simulink library "TMCA_lib"  (Simulink 7.5)
settings: Solver=ode45  StartTime=0.0  StopTime=10.0  RelTol=1e-3
values from neighbouring files (symbols this model uses):
  pTMCA_A_BatCurrHi_C = Simulink.Parameter    [TMCA_par.m]
  pTMCA_A_BatCurrLo_C = Simulink.Parameter    [TMCA_par.m]
  pTMCA_bool_ACPtcConfig_C = Simulink.Parameter    [TMCA_par.m]
  pTMCA_bool_BatCoolACReqCtrl_C = Simulink.Parameter    [TMCA_par.m]
  pTMCA_bool_BatCoolACReqEnbl_C = Simulink.Parameter    [TMCA_par.m]
  pTMCA_bool_BatCoolEnbl_C = Simulink.Parameter    [TMCA_par.m]
  pTMCA_bool_BatHeatEnbl_C = Simulink.Parameter    [TMCA_par.m]
  pTMCA_bool_ChrgrValveCtrl_C = Simulink.Parameter    [TMCA_par.m]
  pTMCA_bool_ChrgrValveEnbl_C = Simulink.Parameter    [TMCA_par.m]
  pTMCA_bool_FanCtrlEnbl = Simulink.Parameter    [TMCA_par.m]
  pTMCA_bool_FanCtrlSwitch = Simulink.Parameter    [TMCA_par.m]
  pTMCA_bool_Mot1PmpEnbl_C = Simulink.Parameter    [TMCA_par.m]
  pTMCA_bool_Mot2PmpEnbl_C = Simulink.Parameter    [TMCA_par.m]
  pTMCA_bool_MotValveCtrl_C = Simulink.Parameter    [TMCA_par.m]
  pTMCA_bool_MotValveEnbl_C = Simulink.Parameter    [TMCA_par.m]
  pTMCA_bool_TMCoolEnbl_C = Simulink.Parameter    [TMCA_par.m]
  pTMCA_bool_WtrPmpCoolEnbl_C = Simulink.Parameter    [TMCA_par.m]
  pTMCA_bool_WtrPmpHeatEnbl_C = Simulink.Parameter    [TMCA_par.m]
  pTMCA_cnt_ACHeatTime_CUR = Simulink.Parameter    [TMCA_par.m]
  pTMCA_cnt_DCTempTime_CUR = Simulink.Parameter    [TMCA_par.m]
  pTMCA_cnt_TimeDwnLim_C = Simulink.Parameter    [TMCA_par.m]
  pTMCA_cnt_TimeUpLim_C = Simulink.Parameter    [TMCA_par.m]
  pTMCA_degC_AmbHiTempDisply_C = Simulink.Parameter    [TMCA_par.m]
  pTMCA_degC_BatCoolAmbHiTemp_C = Simulink.Parameter    [TMCA_par.m]
  pTMCA_degC_BatCoolAmbLoTemp_C = Simulink.Parameter    [TMCA_par.m]
  pTMCA_degC_BatCoolHiTemp_C = Simulink.Parameter    [TMCA_par.m]
  pTMCA_degC_BatCoolLoTemp_C = Simulink.Parameter    [TMCA_par.m]
  pTMCA_degC_BatHiTempDisply_C = Simulink.Parameter    [TMCA_par.m]
  pTMCA_degC_BatMaxT_CUR = Simulink.Parameter    [TMCA_par.m]
  pTMCA_degC_BatMaxTHiThd_C = Simulink.Parameter    [TMCA_par.m]
  pTMCA_degC_BatMaxTLoThd_C = Simulink.Parameter    [TMCA_par.m]
  pTMCA_degC_ChrgrHiTThd_C = Simulink.Parameter    [TMCA_par.m]
  pTMCA_degC_ChrgrLoTThd_C = Simulink.Parameter    [TMCA_par.m]
  pTMCA_degC_ChrgrTThd_CUR = Simulink.Parameter    [TMCA_par.m]
  pTMCA_degC_DcDcHiTThd_C = Simulink.Parameter    [TMCA_par.m]
  pTMCA_degC_DcDcLoTThd_C = Simulink.Parameter    [TMCA_par.m]
  pTMCA_degC_DcDcTThd_CUR = Simulink.Parameter    [TMCA_par.m]
  pTMCA_degC_MotWtrHiTThd_C = Simulink.Parameter    [TMCA_par.m]
  pTMCA_degC_MotWtrLoTThd_C = Simulink.Parameter    [TMCA_par.m]
  pTMCA_degC_MotWtrMaxTThd_C = Simulink.Parameter    [TMCA_par.m]
  pTMCA_degC_MotWtrMinTThd_C = Simulink.Parameter    [TMCA_par.m]
  pTMCA_pct_ACHeatPTCPWM_CUR = Simulink.Parameter    [TMCA_par.m]
  pTMCA_pct_BatWtrPmpPWM_CUR = Simulink.Parameter    [TMCA_par.m]
  pTMCA_pct_ChrgrWtrPmpPWM_CUR = Simulink.Parameter    [TMCA_par.m]
  pTMCA_pct_DcDcWtrPmpPWM_CUR = Simulink.Parameter    [TMCA_par.m]
  pTMCA_pct_DCHeatPTCPWM_CUR = Simulink.Parameter    [TMCA_par.m]
  pTMCA_pct_HeatPTCCtrl_C = Simulink.Parameter    [TMCA_par.m]
  pTMCA_pct_HeatPTCEnbl_C = Simulink.Parameter    [TMCA_par.m]
  pTMCA_pct_HeatrOffVal_C = Simulink.Parameter    [TMCA_par.m]
  pTMCA_pct_Mot1PmpPWMCtrl_C = Simulink.Parameter    [TMCA_par.m]
  pTMCA_pct_Mot2PmpPWMCtrl_C = Simulink.Parameter    [TMCA_par.m]
  pTMCA_pct_MotWtrPmpMaxSpd_C = Simulink.Parameter    [TMCA_par.m]
  pTMCA_pct_MotWtrPmpMinSpd_C = Simulink.Parameter    [TMCA_par.m]
  pTMCA_pct_MotWtrPmpNormSpd_C = Simulink.Parameter    [TMCA_par.m]
  pTMCA_pct_MotWtrPmpZeroSpd_C = Simulink.Parameter    [TMCA_par.m]
  pTMCA_pct_WtrPmpCoolCtrl_C = Simulink.Parameter    [TMCA_par.m]
  pTMCA_pct_WtrPmpHeatCtrl_C = Simulink.Parameter    [TMCA_par.m]
  pTMCA_s_ACDisChrgTimout_C = Simulink.Parameter    [TMCA_par.m]
  pTMCA_s_TFilSampleTi_C = Simulink.Parameter    [TMCA_par.m]
  pTMCA_st_AirCdnOn_C = Simulink.Parameter    [TMCA_par.m]
undefined symbols (not defined in the file or in its folder): AirCdnFanReqTyp, ChrgActStsTyp, MCUCoolReqTyp, p_bool_False_M, p_bool_True_M, PUDCoorrStsTyp
libraries: BaseOperationLib_Browser x197, PES_CZ_FAW x3, simulink x1
(part 2 of 2)

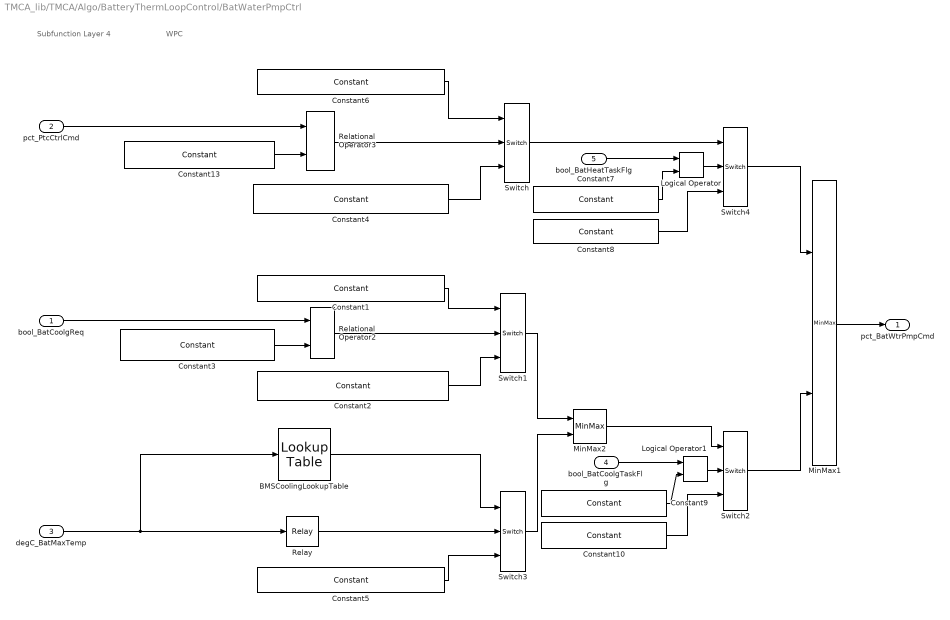
== system TMCA_lib/TMCA/Algo/BatteryThermLoopControl/BatWaterPmpCtrl ==
  note: WPC
  note: Subfunction Layer 4
  bool_BatCoolgReq : Inport  OutDataType=fixdt(1, 16)  OutScaling=2^0
  pct_PtcCtrlCmd : Inport  Port=2  OutDataType=fixdt(1, 16)  OutScaling=2^0
  degC_BatMaxTemp : Inport  Port=3  OutDataType=fixdt(1, 16)  OutScaling=2^0
  bool_BatCoolgTaskFlg : Inport  Port=4  OutDataType=fixdt(1, 16)  OutScaling=2^0
  bool_BatHeatTaskFlg : Inport  Port=5  OutDataType=fixdt(1, 16)  OutScaling=2^0
  BMSCoolingLookupTable : BaseOperationLib_Browser/Lookup Tables Changed/Lookup Table  InputValues=pTMCA_degC_BatMaxT_CUR  Table=pTMCA_pct_BatWtrPmpPWM_CUR  LookUpMeth=Interpolation-Use End Values  OutMin=[]  OutMax=[]  OutDataType=fixdt(1, 16)  OutScaling=2^0  OutDataTypeStr=Inherit: Inherit via back propagation  SaturateOnIntegerOverflow=on
      settings: AttributesFormatString=X:%<InputValues>\nTAB:%<Table>
  Constant1 : BaseOperationLib_Browser/Sources&Sinks/Constant  Value=pTMCA_pct_MotWtrPmpZeroSpd_C  OutMin=[]  OutMax=[]  OutDataType=fixdt(1, 16)  ConRadixGroup=Use specified scaling  OutScaling=2^0  OutDataTypeStr=Inherit: Inherit from 'Constant value'
  Constant10 : BaseOperationLib_Browser/Sources&Sinks/Constant  Value=pTMCA_pct_WtrPmpCoolCtrl_C  OutMin=[]  OutMax=[]  OutDataType=fixdt(1, 16)  ConRadixGroup=Use specified scaling  OutScaling=2^0  OutDataTypeStr=Inherit: Inherit from 'Constant value'
  Constant13 : BaseOperationLib_Browser/Sources&Sinks/Constant  Value=pTMCA_pct_HeatrOffVal_C  OutMin=[]  OutMax=[]  OutDataType=fixdt(1, 16)  ConRadixGroup=Use specified scaling  OutScaling=2^0  OutDataTypeStr=Inherit: Inherit from 'Constant value'
  Constant2 : BaseOperationLib_Browser/Sources&Sinks/Constant  Value=pTMCA_pct_MotWtrPmpMaxSpd_C  OutMin=[]  OutMax=[]  OutDataType=Enum: EgyCoorrStsTyp  ConRadixGroup=Best Precision: Vector-wise  OutScaling=[]  OutDataTypeStr=Inherit: Inherit from 'Constant value'
  Constant3 : BaseOperationLib_Browser/Sources&Sinks/Constant  Value=p_bool_False_M  OutMin=[]  OutMax=[]  OutDataType=fixdt(1, 16)  ConRadixGroup=Use specified scaling  OutScaling=2^0  OutDataTypeStr=Inherit: Inherit from 'Constant value'
  Constant4 : BaseOperationLib_Browser/Sources&Sinks/Constant  Value=pTMCA_pct_MotWtrPmpMaxSpd_C  OutMin=[]  OutMax=[]  OutDataType=Enum: EgyCoorrStsTyp  ConRadixGroup=Best Precision: Vector-wise  OutScaling=[]  OutDataTypeStr=Inherit: Inherit from 'Constant value'
  Constant5 : BaseOperationLib_Browser/Sources&Sinks/Constant  Value=pTMCA_pct_MotWtrPmpZeroSpd_C  OutMin=[]  OutMax=[]  OutDataType=fixdt(1, 16)  ConRadixGroup=Use specified scaling  OutScaling=2^0  OutDataTypeStr=Inherit: Inherit from 'Constant value'
  Constant6 : BaseOperationLib_Browser/Sources&Sinks/Constant  Value=pTMCA_pct_MotWtrPmpZeroSpd_C  OutMin=[]  OutMax=[]  OutDataType=fixdt(1, 16)  ConRadixGroup=Use specified scaling  OutScaling=2^0  OutDataTypeStr=Inherit: Inherit from 'Constant value'
  Constant7 : BaseOperationLib_Browser/Sources&Sinks/Constant  Value=pTMCA_bool_WtrPmpHeatEnbl_C  OutMin=[]  OutMax=[]  OutDataType=fixdt(1, 16)  ConRadixGroup=Use specified scaling  OutScaling=2^0  OutDataTypeStr=Inherit: Inherit from 'Constant value'
  Constant8 : BaseOperationLib_Browser/Sources&Sinks/Constant  Value=pTMCA_pct_WtrPmpHeatCtrl_C  OutMin=[]  OutMax=[]  OutDataType=fixdt(1, 16)  ConRadixGroup=Use specified scaling  OutScaling=2^0  OutDataTypeStr=Inherit: Inherit from 'Constant value'
  Constant9 : BaseOperationLib_Browser/Sources&Sinks/Constant  Value=pTMCA_bool_WtrPmpCoolEnbl_C  OutMin=[]  OutMax=[]  OutDataType=fixdt(1, 16)  ConRadixGroup=Use specified scaling  OutScaling=2^0  OutDataTypeStr=Inherit: Inherit from 'Constant value'
  Logical Operator : BaseOperationLib_Browser/Logic Operations Changed/Logical Operator  Operator=AND  Inputs=2  AllPortsSameDT=on  OutDataTypeMode=Specify via dialog  LogicDataType=PDT_Bool  OutDataTypeStr=PDT_Bool
  Logical Operator1 : BaseOperationLib_Browser/Logic Operations Changed/Logical Operator  Operator=AND  Inputs=2  AllPortsSameDT=on  OutDataTypeMode=Specify via dialog  LogicDataType=PDT_Bool  OutDataTypeStr=PDT_Bool
  MinMax1 : BaseOperationLib_Browser/Math Operations Changed/MinMax  Function=max  Inputs=2  InputSameDT=on  OutMin=[]  OutMax=[]  OutDataType=fixdt(1, 16)  OutScaling=2^0  SaturateOnIntegerOverflow=on
  MinMax2 : BaseOperationLib_Browser/Math Operations Changed/MinMax  Function=max  Inputs=2  InputSameDT=on  OutMin=[]  OutMax=[]  OutDataType=fixdt(1, 16)  OutScaling=2^0  SaturateOnIntegerOverflow=on
  Relational Operator2 : BaseOperationLib_Browser/Logic Operations Changed/Relational Operator  Operator===  InputSameDT=on  LogicOutDataTypeMode=Specify via dialog  LogicDataType=PDT_Bool  OutDataTypeStr=PDT_Bool
  Relational Operator3 : BaseOperationLib_Browser/Logic Operations Changed/Relational Operator  Operator===  InputSameDT=on  LogicOutDataTypeMode=Specify via dialog  LogicDataType=PDT_Bool  OutDataTypeStr=PDT_Bool
  Relay : BaseOperationLib_Browser/Discontinuities Changed/Relay  OnSwitchValue=pTMCA_degC_BatMaxTHiThd_C  OffSwitchValue=pTMCA_degC_BatMaxTLoThd_C  OnOutputValue=p_bool_True_M  OffOutputValue=p_bool_False_M  OutMin=[]  OutMax=[]  OutDataType=fixdt(1, 16)  ConRadixGroup=Use specified scaling  OutScaling=2^0  OutDataTypeStr=Inherit: Inherit via back propagation
      settings: AttributesFormatString=%<OnSwitchValue> OnOut %<OnOutputValue>\n%<OffSwitchValue> OffOut %<OffOutputValue>
  Switch{,1..4} (5 alike) : BaseOperationLib_Browser/Signal Routing Changed/Switch  Criteria=u2 ~= 0  Threshold=1  InputSameDT=on  OutMin=[]  OutMax=[]  OutDataType=fixdt(1,16,0)  OutScaling=[]  SaturateOnIntegerOverflow=on
  pct_BatWtrPmpCmd : Outport  OutDataType=fixdt(1, 16)  OutScaling=2^0
  wires:
  Constant2/1 -> Switch1/3
  Constant1/1 -> Switch1/1
  Relational Operator2/1 -> Switch1/2
  bool_BatCoolgReq/1 -> Relational Operator2/1
  Constant3/1 -> Relational Operator2/2
  Constant6/1 -> Switch/1
  Constant4/1 -> Switch/3
  Relational Operator3/1 -> Switch/2
  Constant13/1 -> Relational Operator3/2
  pct_PtcCtrlCmd/1 -> Relational Operator3/1
  Switch/1 -> Switch4/1
  Relay/1 -> Switch3/2
  degC_BatMaxTemp/1 -> Relay/1, BMSCoolingLookupTable/1
  BMSCoolingLookupTable/1 -> Switch3/1
  Constant5/1 -> Switch3/3
  Switch1/1 -> MinMax2/1
  Switch3/1 -> MinMax2/2
  MinMax2/1 -> Switch2/1
  Switch4/1 -> MinMax1/1
  Switch2/1 -> MinMax1/2
  MinMax1/1 -> pct_BatWtrPmpCmd/1
  Logical Operator/1 -> Switch4/2
  bool_BatHeatTaskFlg/1 -> Logical Operator/1
  Logical Operator1/1 -> Switch2/2
  bool_BatCoolgTaskFlg/1 -> Logical Operator1/1
  Constant7/1 -> Logical Operator/2
  Constant8/1 -> Switch4/3
  Constant9/1 -> Logical Operator1/2
  Constant10/1 -> Switch2/3

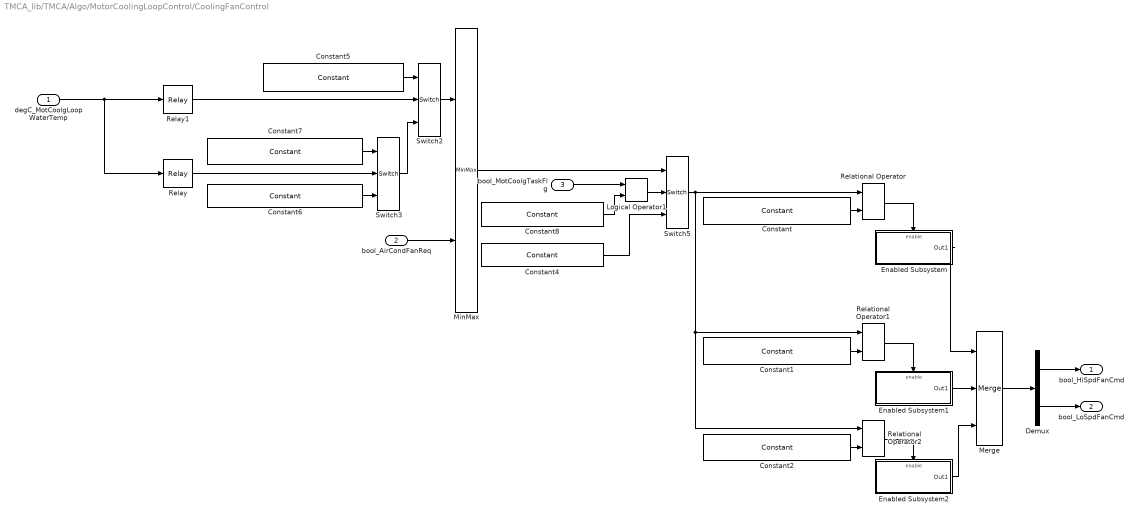
== system TMCA_lib/TMCA/Algo/MotorCoolingLoopControl/CoolingFanControl ==
  degC_MotCoolgLoopWaterTemp : Inport  OutDataType=fixdt(1, 16)  OutScaling=2^0
  bool_AirCondFanReq : Inport  Port=2  OutDataType=fixdt(1, 16)  OutScaling=2^0
  bool_MotCoolgTaskFlg : Inport  Port=3  OutDataType=fixdt(1, 16)  OutScaling=2^0
  Constant : BaseOperationLib_Browser/Sources&Sinks/Constant  Value=uint8(AirCdnFanReqTyp.ACF_HI_SPD)  OutMin=[]  OutMax=[]  OutDataType=fixdt(1, 16)  ConRadixGroup=Use specified scaling  OutScaling=2^0  OutDataTypeStr=Inherit: Inherit from 'Constant value'
  Constant1 : BaseOperationLib_Browser/Sources&Sinks/Constant  Value=uint8(AirCdnFanReqTyp.ACF_LO_SPD)  OutMin=[]  OutMax=[]  OutDataType=fixdt(1, 16)  ConRadixGroup=Use specified scaling  OutScaling=2^0  OutDataTypeStr=Inherit: Inherit from 'Constant value'
  Constant2 : BaseOperationLib_Browser/Sources&Sinks/Constant  Value=uint8(AirCdnFanReqTyp.ACF_OFF)  OutMin=[]  OutMax=[]  OutDataType=fixdt(1, 16)  ConRadixGroup=Use specified scaling  OutScaling=2^0  OutDataTypeStr=Inherit: Inherit from 'Constant value'
  Constant4 : BaseOperationLib_Browser/Sources&Sinks/Constant  Value=pTMCA_bool_FanCtrlSwitch  OutMin=[]  OutMax=[]  OutDataType=fixdt(1, 16)  ConRadixGroup=Use specified scaling  OutScaling=2^0  OutDataTypeStr=Inherit: Inherit from 'Constant value'
  Constant5 : BaseOperationLib_Browser/Sources&Sinks/Constant  Value=uint8(AirCdnFanReqTyp.ACF_HI_SPD)  OutMin=[]  OutMax=[]  OutDataType=fixdt(1, 16)  ConRadixGroup=Use specified scaling  OutScaling=2^0  OutDataTypeStr=Inherit: Inherit from 'Constant value'
  Constant6 : BaseOperationLib_Browser/Sources&Sinks/Constant  Value=uint8(AirCdnFanReqTyp.ACF_OFF)  OutMin=[]  OutMax=[]  OutDataType=fixdt(1, 16)  ConRadixGroup=Use specified scaling  OutScaling=2^0  OutDataTypeStr=Inherit: Inherit from 'Constant value'
  Constant7 : BaseOperationLib_Browser/Sources&Sinks/Constant  Value=uint8(AirCdnFanReqTyp.ACF_LO_SPD)  OutMin=[]  OutMax=[]  OutDataType=fixdt(1, 16)  ConRadixGroup=Use specified scaling  OutScaling=2^0  OutDataTypeStr=Inherit: Inherit from 'Constant value'
  Constant8 : BaseOperationLib_Browser/Sources&Sinks/Constant  Value=pTMCA_bool_FanCtrlEnbl  OutMin=[]  OutMax=[]  OutDataType=fixdt(1, 16)  ConRadixGroup=Use specified scaling  OutScaling=2^0  OutDataTypeStr=Inherit: Inherit from 'Constant value'
  Demux : Demux  Outputs=2
  Enabled Subsystem : Subsystem  TreatAsAtomicUnit=on
  Enabled Subsystem1 : Subsystem  TreatAsAtomicUnit=on
  Enabled Subsystem2 : Subsystem  TreatAsAtomicUnit=on
  Logical Operator1 : BaseOperationLib_Browser/Logic Operations Changed/Logical Operator  Operator=AND  Inputs=2  AllPortsSameDT=on  OutDataTypeMode=Specify via dialog  LogicDataType=PDT_Bool  OutDataTypeStr=PDT_Bool
  Merge : Merge  Inputs=3
  MinMax : BaseOperationLib_Browser/Math Operations Changed/MinMax  Function=max  Inputs=2  InputSameDT=on  OutMin=[]  OutMax=[]  OutDataTypeMode=uint8  OutDataType=fixdt(1, 16)  OutScaling=2^0  OutDataTypeStr=uint8  SaturateOnIntegerOverflow=on
  Relational Operator : BaseOperationLib_Browser/Logic Operations Changed/Relational Operator  Operator===  InputSameDT=on  LogicOutDataTypeMode=Specify via dialog  LogicDataType=PDT_Bool  OutDataTypeStr=PDT_Bool
  Relational Operator1 : BaseOperationLib_Browser/Logic Operations Changed/Relational Operator  Operator===  InputSameDT=on  LogicOutDataTypeMode=Specify via dialog  LogicDataType=PDT_Bool  OutDataTypeStr=PDT_Bool
  Relational Operator2 : BaseOperationLib_Browser/Logic Operations Changed/Relational Operator  Operator===  InputSameDT=on  LogicOutDataTypeMode=Specify via dialog  LogicDataType=PDT_Bool  OutDataTypeStr=PDT_Bool
  Relay : BaseOperationLib_Browser/Discontinuities Changed/Relay  OnSwitchValue=pTMCA_degC_MotWtrHiTThd_C  OffSwitchValue=pTMCA_degC_MotWtrLoTThd_C  OnOutputValue=p_bool_True_M  OffOutputValue=p_bool_False_M  OutMin=[]  OutMax=[]  OutDataType=fixdt(1, 16)  ConRadixGroup=Use specified scaling  OutScaling=2^0  OutDataTypeStr=Inherit: Inherit via back propagation
      settings: AttributesFormatString=%<OnSwitchValue> OnOut %<OnOutputValue>\n%<OffSwitchValue> OffOut %<OffOutputValue>
  Relay1 : BaseOperationLib_Browser/Discontinuities Changed/Relay  OnSwitchValue=pTMCA_degC_MotWtrMaxTThd_C  OffSwitchValue=pTMCA_degC_MotWtrMinTThd_C  OnOutputValue=p_bool_True_M  OffOutputValue=p_bool_False_M  OutMin=[]  OutMax=[]  OutDataType=fixdt(1, 16)  ConRadixGroup=Use specified scaling  OutScaling=2^0  OutDataTypeStr=Inherit: Inherit via back propagation
      settings: AttributesFormatString=%<OnSwitchValue> OnOut %<OnOutputValue>\n%<OffSwitchValue> OffOut %<OffOutputValue>
  Switch2 : BaseOperationLib_Browser/Signal Routing Changed/Switch  Criteria=u2 ~= 0  Threshold=1  InputSameDT=on  OutMin=[]  OutMax=[]  OutDataType=fixdt(1,16,0)  OutScaling=[]  SaturateOnIntegerOverflow=on
  Switch3 : BaseOperationLib_Browser/Signal Routing Changed/Switch  Criteria=u2 ~= 0  Threshold=1  InputSameDT=on  OutMin=[]  OutMax=[]  OutDataType=fixdt(1,16,0)  OutScaling=[]  SaturateOnIntegerOverflow=on
  Switch5 : BaseOperationLib_Browser/Signal Routing Changed/Switch  Criteria=u2 ~= 0  Threshold=1  InputSameDT=on  OutMin=[]  OutMax=[]  OutDataType=fixdt(1,16,0)  OutScaling=[]  SaturateOnIntegerOverflow=on
  bool_HiSpdFanCmd : Outport  OutDataType=fixdt(1, 16)  OutScaling=2^0
  bool_LoSpdFanCmd : Outport  Port=2  OutDataType=fixdt(1, 16)  OutScaling=2^0
  wires:
  Merge/1 -> Demux/1
  Enabled Subsystem2/1(Out1) -> Merge/3
  Enabled Subsystem1/1(Out1) -> Merge/2
  Demux/2 -> bool_LoSpdFanCmd/1
  Demux/1 -> bool_HiSpdFanCmd/1
  Enabled Subsystem/1(Out1) -> Merge/1
  Relational Operator2/1 -> Enabled Subsystem2/Enable
  Relational Operator1/1 -> Enabled Subsystem1/Enable
  Relational Operator/1 -> Enabled Subsystem/Enable
  Constant2/1 -> Relational Operator2/2
  Switch5/1 -> Relational Operator2/1, Relational Operator1/1, Relational Operator/1
  Constant4/1 -> Switch5/3
  Constant8/1 -> Logical Operator1/2
  MinMax/1 -> Switch5/1
  bool_MotCoolgTaskFlg/1 -> Logical Operator1/1
  Logical Operator1/1 -> Switch5/2
  bool_AirCondFanReq/1 -> MinMax/2
  Relay1/1 -> Switch2/2
  degC_MotCoolgLoopWaterTemp/1 -> Relay1/1, Relay/1
  Constant1/1 -> Relational Operator1/2
  Constant/1 -> Relational Operator/2
  Relay/1 -> Switch3/2
  Constant6/1 -> Switch3/3
  Constant7/1 -> Switch3/1
  Switch3/1 -> Switch2/3
  Constant5/1 -> Switch2/1
  Switch2/1 -> MinMax/1

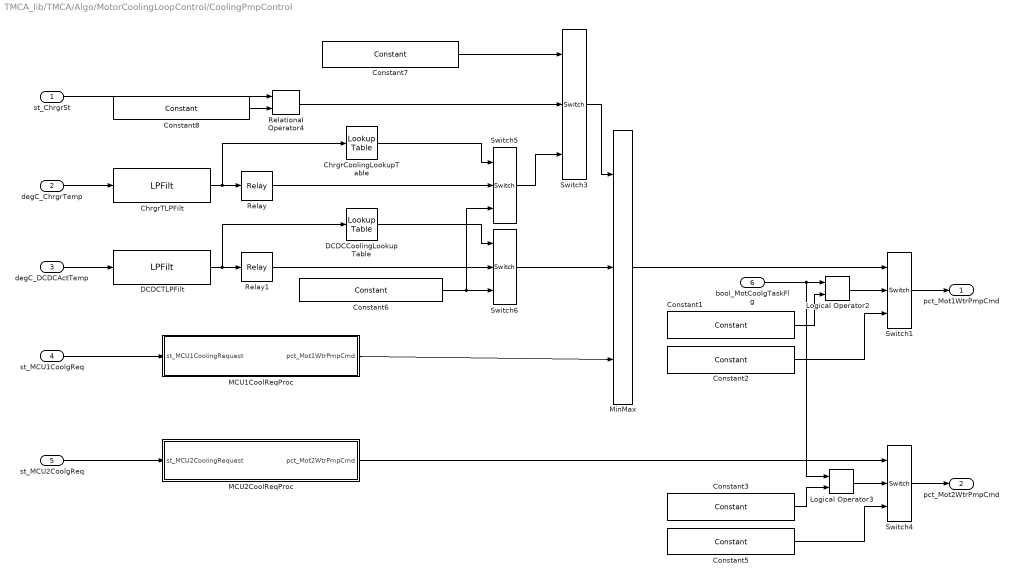
== system TMCA_lib/TMCA/Algo/MotorCoolingLoopControl/CoolingPmpControl ==
  st_ChrgrSt : Inport  OutDataType=fixdt(1, 16)  OutScaling=2^0
  degC_ChrgrTemp : Inport  Port=2  OutDataType=fixdt(1, 16)  OutScaling=2^0
  degC_DCDCActTemp : Inport  Port=3  OutDataType=fixdt(1, 16)  OutScaling=2^0
  st_MCU1CoolgReq : Inport  Port=4  OutDataType=fixdt(1, 16)  OutScaling=2^0
  st_MCU2CoolgReq : Inport  Port=5  OutDataType=fixdt(1, 16)  OutScaling=2^0
  bool_MotCoolgTaskFlg : Inport  Port=6  OutDataType=fixdt(1, 16)  OutScaling=2^0
  ChrgrCoolingLookupTable : BaseOperationLib_Browser/Lookup Tables Changed/Lookup Table  InputValues=pTMCA_degC_ChrgrTThd_CUR  Table=pTMCA_pct_ChrgrWtrPmpPWM_CUR  LookUpMeth=Interpolation-Use End Values  OutMin=[]  OutMax=[]  OutDataType=fixdt(1, 16)  OutScaling=2^0  OutDataTypeStr=Inherit: Inherit via back propagation  SaturateOnIntegerOverflow=on
      settings: AttributesFormatString=X:%<InputValues>\nTAB:%<Table>
  ChrgrTLPFilt : PES_CZ_FAW/Filters/LPFilt  SystemSampleTime=-1  Ts=pTMCA_s_TFilSampleTi_C  Tau=pTMCA_s_TFilTau_C
      settings: FunctionWithSeparateData=on
  Constant1 : BaseOperationLib_Browser/Sources&Sinks/Constant  Value=pTMCA_bool_Mot1PmpEnbl_C  OutMin=[]  OutMax=[]  OutDataType=fixdt(1, 16)  ConRadixGroup=Use specified scaling  OutScaling=2^0  OutDataTypeStr=Inherit: Inherit from 'Constant value'
  Constant2 : BaseOperationLib_Browser/Sources&Sinks/Constant  Value=pTMCA_pct_Mot1PmpPWMCtrl_C  OutMin=[]  OutMax=[]  OutDataType=fixdt(1, 16)  ConRadixGroup=Use specified scaling  OutScaling=2^0  OutDataTypeStr=Inherit: Inherit from 'Constant value'
  Constant3 : BaseOperationLib_Browser/Sources&Sinks/Constant  Value=pTMCA_bool_Mot2PmpEnbl_C  OutMin=[]  OutMax=[]  OutDataType=fixdt(1, 16)  ConRadixGroup=Use specified scaling  OutScaling=2^0  OutDataTypeStr=Inherit: Inherit from 'Constant value'
  Constant5 : BaseOperationLib_Browser/Sources&Sinks/Constant  Value=pTMCA_pct_Mot2PmpPWMCtrl_C  OutMin=[]  OutMax=[]  OutDataType=fixdt(1, 16)  ConRadixGroup=Use specified scaling  OutScaling=2^0  OutDataTypeStr=Inherit: Inherit from 'Constant value'
  Constant6 : BaseOperationLib_Browser/Sources&Sinks/Constant  Value=pTMCA_pct_MotWtrPmpZeroSpd_C  OutMin=[]  OutMax=[]  OutDataType=fixdt(1, 16)  ConRadixGroup=Use specified scaling  OutScaling=2^0  OutDataTypeStr=Inherit: Inherit from 'Constant value'
  Constant7 : BaseOperationLib_Browser/Sources&Sinks/Constant  Value=pTMCA_pct_MotWtrPmpZeroSpd_C  OutMin=[]  OutMax=[]  OutDataType=fixdt(1, 16)  ConRadixGroup=Use specified scaling  OutScaling=2^0  OutDataTypeStr=Inherit: Inherit from 'Constant value'
  Constant8 : BaseOperationLib_Browser/Sources&Sinks/Constant  Value=uint8(ChrgActStsTyp.IDLE)  OutMin=[]  OutMax=[]  OutDataType=fixdt(1, 16)  ConRadixGroup=Use specified scaling  OutScaling=2^0  OutDataTypeStr=Inherit: Inherit from 'Constant value'
  DCDCCoolingLookupTable : BaseOperationLib_Browser/Lookup Tables Changed/Lookup Table  InputValues=pTMCA_degC_DcDcTThd_CUR  Table=pTMCA_pct_DcDcWtrPmpPWM_CUR  LookUpMeth=Interpolation-Use End Values  OutMin=[]  OutMax=[]  OutDataType=fixdt(1, 16)  OutScaling=2^0  OutDataTypeStr=Inherit: Inherit via back propagation  SaturateOnIntegerOverflow=on
      settings: AttributesFormatString=X:%<InputValues>\nTAB:%<Table>
  DCDCTLPFilt : PES_CZ_FAW/Filters/LPFilt  SystemSampleTime=-1  Ts=pTMCA_s_TFilSampleTi_C  Tau=pTMCA_s_TFilTau_C
      settings: FunctionWithSeparateData=on
  Logical Operator2 : BaseOperationLib_Browser/Logic Operations Changed/Logical Operator  Operator=AND  Inputs=2  AllPortsSameDT=on  OutDataTypeMode=Specify via dialog  LogicDataType=PDT_Bool  OutDataTypeStr=PDT_Bool
  Logical Operator3 : BaseOperationLib_Browser/Logic Operations Changed/Logical Operator  Operator=AND  Inputs=2  AllPortsSameDT=on  OutDataTypeMode=Specify via dialog  LogicDataType=PDT_Bool  OutDataTypeStr=PDT_Bool
  MCU1CoolReqProc : Subsystem
  MCU2CoolReqProc : Subsystem
  MinMax : BaseOperationLib_Browser/Math Operations Changed/MinMax  Function=max  Inputs=3  InputSameDT=on  OutMin=[]  OutMax=[]  OutDataType=fixdt(1, 16)  OutScaling=2^0  SaturateOnIntegerOverflow=on
  Relational Operator4 : BaseOperationLib_Browser/Logic Operations Changed/Relational Operator  Operator===  InputSameDT=on  LogicOutDataTypeMode=Specify via dialog  LogicDataType=PDT_Bool  OutDataTypeStr=PDT_Bool
  Relay : BaseOperationLib_Browser/Discontinuities Changed/Relay  OnSwitchValue=pTMCA_degC_ChrgrHiTThd_C  OffSwitchValue=pTMCA_degC_ChrgrLoTThd_C  OnOutputValue=p_bool_True_M  OffOutputValue=p_bool_False_M  OutMin=[]  OutMax=[]  OutDataType=fixdt(1, 16)  ConRadixGroup=Use specified scaling  OutScaling=2^0  OutDataTypeStr=Inherit: Inherit via back propagation
      settings: AttributesFormatString=%<OnSwitchValue> OnOut %<OnOutputValue>\n%<OffSwitchValue> OffOut %<OffOutputValue>
  Relay1 : BaseOperationLib_Browser/Discontinuities Changed/Relay  OnSwitchValue=pTMCA_degC_DcDcHiTThd_C  OffSwitchValue=pTMCA_degC_DcDcLoTThd_C  OnOutputValue=p_bool_True_M  OffOutputValue=p_bool_False_M  OutMin=[]  OutMax=[]  OutDataType=fixdt(1, 16)  ConRadixGroup=Use specified scaling  OutScaling=2^0  OutDataTypeStr=Inherit: Inherit via back propagation
      settings: AttributesFormatString=%<OnSwitchValue> OnOut %<OnOutputValue>\n%<OffSwitchValue> OffOut %<OffOutputValue>
  Switch{1,3..6} (5 alike) : BaseOperationLib_Browser/Signal Routing Changed/Switch  Criteria=u2 ~= 0  Threshold=1  InputSameDT=on  OutMin=[]  OutMax=[]  OutDataType=fixdt(1,16,0)  OutScaling=[]  SaturateOnIntegerOverflow=on
  pct_Mot1WtrPmpCmd : Outport  OutDataType=fixdt(1, 16)  OutScaling=2^0
  pct_Mot2WtrPmpCmd : Outport  Port=2  OutDataType=fixdt(1, 16)  OutScaling=2^0
  wires:
  MCU2CoolReqProc/1(pct_Mot2WtrPmpCmd) -> Switch4/1
  st_MCU1CoolgReq/1 -> MCU1CoolReqProc/1(st_MCU1CoolingRequest)
  degC_ChrgrTemp/1 -> ChrgrTLPFilt/1
  degC_DCDCActTemp/1 -> DCDCTLPFilt/1
  MCU1CoolReqProc/1(pct_Mot1WtrPmpCmd) -> MinMax/3
  st_MCU2CoolgReq/1 -> MCU2CoolReqProc/1(st_MCU2CoolingRequest)
  MinMax/1 -> Switch1/1
  st_ChrgrSt/1 -> Relational Operator4/1
  Relational Operator4/1 -> Switch3/2
  Constant7/1 -> Switch3/1
  Switch3/1 -> MinMax/1
  Constant8/1 -> Relational Operator4/2
  Switch1/1 -> pct_Mot1WtrPmpCmd/1
  Switch4/1 -> pct_Mot2WtrPmpCmd/1
  Constant2/1 -> Switch1/3
  Constant5/1 -> Switch4/3
  ChrgrTLPFilt/1 -> Relay/1, ChrgrCoolingLookupTable/1
  Switch5/1 -> Switch3/3
  ChrgrCoolingLookupTable/1 -> Switch5/1
  Switch6/1 -> MinMax/2
  Relay1/1 -> Switch6/2
  DCDCTLPFilt/1 -> Relay1/1, DCDCCoolingLookupTable/1
  DCDCCoolingLookupTable/1 -> Switch6/1
  Relay/1 -> Switch5/2
  Constant6/1 -> Switch6/3, Switch5/3
  Logical Operator2/1 -> Switch1/2
  bool_MotCoolgTaskFlg/1 -> Logical Operator2/1, Logical Operator3/1
  Logical Operator3/1 -> Switch4/2
  Constant1/1 -> Logical Operator2/2
  Constant3/1 -> Logical Operator3/2

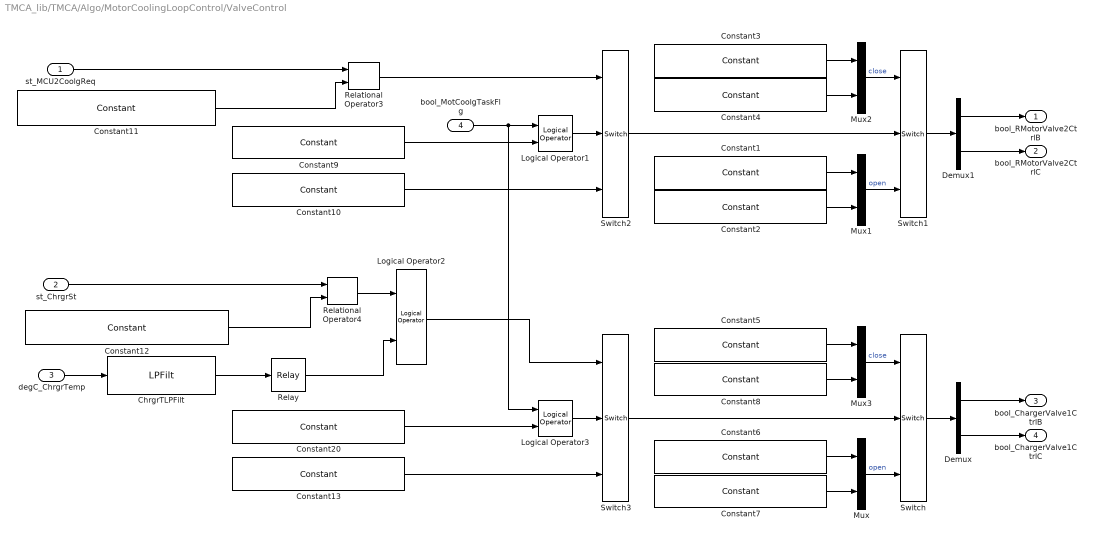
== system TMCA_lib/TMCA/Algo/MotorCoolingLoopControl/ValveControl ==
  st_MCU2CoolgReq : Inport
  st_ChrgrSt : Inport  Port=2  OutDataType=fixdt(1, 16)  OutScaling=2^0
  degC_ChrgrTemp : Inport  Port=3  OutDataType=fixdt(1, 16)  OutScaling=2^0
  bool_MotCoolgTaskFlg : Inport  Port=4
  ChrgrTLPFilt : PES_CZ_FAW/Filters/LPFilt  SystemSampleTime=-1  Ts=pTMCA_s_TFilSampleTi_C  Tau=pTMCA_s_TFilTau_C
      settings: FunctionWithSeparateData=on
  Constant{1,4,6,8} (4 alike) : BaseOperationLib_Browser/Sources&Sinks/Constant  Value=p_bool_True_M  OutMin=[]  OutMax=[]  OutDataType=fixdt(1, 16)  ConRadixGroup=Use specified scaling  OutScaling=2^0  OutDataTypeStr=Inherit: Inherit from 'Constant value'
  Constant10 : BaseOperationLib_Browser/Sources&Sinks/Constant  Value=pTMCA_bool_MotValveCtrl_C  OutMin=[]  OutMax=[]  OutDataType=fixdt(1, 16)  ConRadixGroup=Use specified scaling  OutScaling=2^0  OutDataTypeStr=Inherit: Inherit from 'Constant value'
  Constant11 : BaseOperationLib_Browser/Sources&Sinks/Constant  Value=uint8(MCUCoolReqTyp.MCU_NoFlowReq)  OutMin=[]  OutMax=[]  OutDataType=fixdt(1, 16)  ConRadixGroup=Use specified scaling  OutScaling=2^0  OutDataTypeStr=Inherit: Inherit from 'Constant value'
  Constant12 : BaseOperationLib_Browser/Sources&Sinks/Constant  Value=uint8(ChrgActStsTyp.IDLE)  OutMin=[]  OutMax=[]  OutDataType=fixdt(1, 16)  ConRadixGroup=Use specified scaling  OutScaling=2^0  OutDataTypeStr=Inherit: Inherit from 'Constant value'
  Constant13 : BaseOperationLib_Browser/Sources&Sinks/Constant  Value=pTMCA_bool_ChrgrValveCtrl_C  OutMin=[]  OutMax=[]  OutDataType=fixdt(1, 16)  ConRadixGroup=Use specified scaling  OutScaling=2^0  OutDataTypeStr=Inherit: Inherit from 'Constant value'
  Constant{2..3,5,7} (4 alike) : BaseOperationLib_Browser/Sources&Sinks/Constant  Value=p_bool_False_M  OutMin=[]  OutMax=[]  OutDataType=fixdt(1, 16)  ConRadixGroup=Use specified scaling  OutScaling=2^0  OutDataTypeStr=Inherit: Inherit from 'Constant value'
  Constant20 : BaseOperationLib_Browser/Sources&Sinks/Constant  Value=pTMCA_bool_ChrgrValveEnbl_C  OutMin=[]  OutMax=[]  OutDataType=fixdt(1, 16)  ConRadixGroup=Use specified scaling  OutScaling=2^0  OutDataTypeStr=Inherit: Inherit from 'Constant value'
  Constant9 : BaseOperationLib_Browser/Sources&Sinks/Constant  Value=pTMCA_bool_MotValveEnbl_C  OutMin=[]  OutMax=[]  OutDataType=fixdt(1, 16)  ConRadixGroup=Use specified scaling  OutScaling=2^0  OutDataTypeStr=Inherit: Inherit from 'Constant value'
  Demux : Demux  Outputs=2
  Demux1 : Demux  Outputs=2
  Logical Operator1 : BaseOperationLib_Browser/Logic Operations Changed/Logical Operator  Operator=AND  Inputs=2  AllPortsSameDT=on  OutDataTypeMode=Specify via dialog  LogicDataType=PDT_Bool  OutDataTypeStr=PDT_Bool
  Logical Operator2 : BaseOperationLib_Browser/Logic Operations Changed/Logical Operator  Operator=AND  Inputs=2  AllPortsSameDT=on  OutDataTypeMode=Specify via dialog  LogicDataType=PDT_Bool  OutDataTypeStr=PDT_Bool
  Logical Operator3 : BaseOperationLib_Browser/Logic Operations Changed/Logical Operator  Operator=AND  Inputs=2  AllPortsSameDT=on  OutDataTypeMode=Specify via dialog  LogicDataType=PDT_Bool  OutDataTypeStr=PDT_Bool
  Mux{,1..3} (4 alike) : Mux  Inputs=2
  Relational Operator3 : BaseOperationLib_Browser/Logic Operations Changed/Relational Operator  Operator===  InputSameDT=on  LogicOutDataTypeMode=Specify via dialog  LogicDataType=PDT_Bool  OutDataTypeStr=PDT_Bool
  Relational Operator4 : BaseOperationLib_Browser/Logic Operations Changed/Relational Operator  Operator=~=  InputSameDT=on  LogicOutDataTypeMode=Specify via dialog  LogicDataType=PDT_Bool  OutDataTypeStr=PDT_Bool
  Relay : BaseOperationLib_Browser/Discontinuities Changed/Relay  OnSwitchValue=pTMCA_degC_ChrgrHiTThd_C  OffSwitchValue=pTMCA_degC_ChrgrLoTThd_C  OnOutputValue=p_bool_True_M  OffOutputValue=p_bool_False_M  OutMin=[]  OutMax=[]  OutDataType=fixdt(1, 16)  ConRadixGroup=Use specified scaling  OutScaling=2^0  OutDataTypeStr=Inherit: Inherit via back propagation
      settings: AttributesFormatString=%<OnSwitchValue> OnOut %<OnOutputValue>\n%<OffSwitchValue> OffOut %<OffOutputValue>
  Switch{,1..3} (4 alike) : BaseOperationLib_Browser/Signal Routing Changed/Switch  Criteria=u2 ~= 0  Threshold=1  InputSameDT=on  OutMin=[]  OutMax=[]  OutDataType=fixdt(1,16,0)  OutScaling=[]  SaturateOnIntegerOverflow=on
  bool_RMotorValve2CtrlB : Outport
  bool_RMotorValve2CtrlC : Outport  Port=2
  bool_ChargerValve1CtrlB : Outport  Port=3
  bool_ChargerValve1CtrlC : Outport  Port=4
  wires:
  Mux3/1 -> Switch/1  "close"
  Mux/1 -> Switch/3  "open"
  Mux1/1 -> Switch1/3  "open"
  Mux2/1 -> Switch1/1  "close"
  Constant4/1 -> Mux2/2
  Constant3/1 -> Mux2/1
  Demux1/2 -> bool_RMotorValve2CtrlC/1
  Demux1/1 -> bool_RMotorValve2CtrlB/1
  Switch1/1 -> Demux1/1
  Constant2/1 -> Mux1/2
  Constant1/1 -> Mux1/1
  Constant8/1 -> Mux3/2
  Constant5/1 -> Mux3/1
  Demux/2 -> bool_ChargerValve1CtrlC/1
  Demux/1 -> bool_ChargerValve1CtrlB/1
  Switch/1 -> Demux/1
  Constant7/1 -> Mux/2
  Constant6/1 -> Mux/1
  Constant11/1 -> Relational Operator3/2
  st_MCU2CoolgReq/1 -> Relational Operator3/1
  Constant12/1 -> Relational Operator4/2
  st_ChrgrSt/1 -> Relational Operator4/1
  Relational Operator4/1 -> Logical Operator2/1
  degC_ChrgrTemp/1 -> ChrgrTLPFilt/1
  Relay/1 -> Logical Operator2/2
  ChrgrTLPFilt/1 -> Relay/1
  Switch2/1 -> Switch1/2
  Relational Operator3/1 -> Switch2/1
  Switch3/1 -> Switch/2
  Logical Operator2/1 -> Switch3/1
  Logical Operator1/1 -> Switch2/2
  Logical Operator3/1 -> Switch3/2
  bool_MotCoolgTaskFlg/1 -> Logical Operator1/1, Logical Operator3/1
  Constant9/1 -> Logical Operator1/2
  Constant10/1 -> Switch2/3
  Constant20/1 -> Logical Operator3/2
  Constant13/1 -> Switch3/3

== system TMCA_lib/TMCA/Algo/MotorCoolingLoopControl/CoolingFanControl/Enabled Subsystem ==
  Enable : EnablePort
  Constant1 : BaseOperationLib_Browser/Sources&Sinks/Constant  Value=p_bool_True_M  OutMin=[]  OutMax=[]  OutDataType=fixdt(1, 16)  ConRadixGroup=Use specified scaling  OutScaling=2^0  OutDataTypeStr=Inherit: Inherit from 'Constant value'
  Constant2 : BaseOperationLib_Browser/Sources&Sinks/Constant  Value=p_bool_True_M  OutMin=[]  OutMax=[]  OutDataType=fixdt(1, 16)  ConRadixGroup=Use specified scaling  OutScaling=2^0  OutDataTypeStr=Inherit: Inherit from 'Constant value'
  Mux1 : Mux  Inputs=2
  Out1 : Outport  OutDataType=fixdt(1, 16)  OutScaling=2^0
  wires:
  Mux1/1 -> Out1/1
  Constant2/1 -> Mux1/2
  Constant1/1 -> Mux1/1

== system TMCA_lib/TMCA/Algo/MotorCoolingLoopControl/CoolingFanControl/Enabled Subsystem1 ==
  Enable : EnablePort
  Constant3 : BaseOperationLib_Browser/Sources&Sinks/Constant  Value=p_bool_False_M  OutMin=[]  OutMax=[]  OutDataType=fixdt(1, 16)  ConRadixGroup=Use specified scaling  OutScaling=2^0  OutDataTypeStr=Inherit: Inherit from 'Constant value'
  Constant4 : BaseOperationLib_Browser/Sources&Sinks/Constant  Value=p_bool_True_M  OutMin=[]  OutMax=[]  OutDataType=fixdt(1, 16)  ConRadixGroup=Use specified scaling  OutScaling=2^0  OutDataTypeStr=Inherit: Inherit from 'Constant value'
  Mux2 : Mux  Inputs=2
  Out1 : Outport  OutDataType=fixdt(1, 16)  OutScaling=2^0
  wires:
  Constant4/1 -> Mux2/2
  Constant3/1 -> Mux2/1
  Mux2/1 -> Out1/1

== system TMCA_lib/TMCA/Algo/MotorCoolingLoopControl/CoolingFanControl/Enabled Subsystem2 ==
  Enable : EnablePort
  Constant1 : BaseOperationLib_Browser/Sources&Sinks/Constant  Value=p_bool_False_M  OutMin=[]  OutMax=[]  OutDataType=fixdt(1, 16)  ConRadixGroup=Use specified scaling  OutScaling=2^0  OutDataTypeStr=Inherit: Inherit from 'Constant value'
  Constant2 : BaseOperationLib_Browser/Sources&Sinks/Constant  Value=p_bool_False_M  OutMin=[]  OutMax=[]  OutDataType=fixdt(1, 16)  ConRadixGroup=Use specified scaling  OutScaling=2^0  OutDataTypeStr=Inherit: Inherit from 'Constant value'
  Mux1 : Mux  Inputs=2
  Out1 : Outport  OutDataType=fixdt(1, 16)  OutScaling=2^0
  wires:
  Mux1/1 -> Out1/1
  Constant2/1 -> Mux1/2
  Constant1/1 -> Mux1/1

== system TMCA_lib/TMCA/Algo/MotorCoolingLoopControl/CoolingPmpControl/MCU1CoolReqProc ==
  st_MCU1CoolingRequest : Inport  OutDataType=fixdt(1, 16)  OutScaling=2^0
  Constant : BaseOperationLib_Browser/Sources&Sinks/Constant  Value=uint8(MCUCoolReqTyp.MCU_MaxFlowReq)  OutMin=[]  OutMax=[]  OutDataType=fixdt(1, 16)  ConRadixGroup=Use specified scaling  OutScaling=2^0  OutDataTypeStr=Inherit: Inherit from 'Constant value'
  Constant1 : BaseOperationLib_Browser/Sources&Sinks/Constant  Value=uint8(MCUCoolReqTyp.MCU_MinFlowReq)  OutMin=[]  OutMax=[]  OutDataType=fixdt(1, 16)  ConRadixGroup=Use specified scaling  OutScaling=2^0  OutDataTypeStr=Inherit: Inherit from 'Constant value'
  Constant2 : BaseOperationLib_Browser/Sources&Sinks/Constant  Value=pTMCA_pct_MotWtrPmpZeroSpd_C  OutMin=[]  OutMax=[]  OutDataType=fixdt(1, 16)  ConRadixGroup=Use specified scaling  OutScaling=2^0  OutDataTypeStr=Inherit: Inherit from 'Constant value'
  Constant3 : BaseOperationLib_Browser/Sources&Sinks/Constant  Value=pTMCA_pct_MotWtrPmpMaxSpd_C  OutMin=[]  OutMax=[]  OutDataType=fixdt(1, 16)  ConRadixGroup=Use specified scaling  OutScaling=2^0  OutDataTypeStr=Inherit: Inherit from 'Constant value'
  Constant4 : BaseOperationLib_Browser/Sources&Sinks/Constant  Value=pTMCA_pct_MotWtrPmpMinSpd_C  OutMin=[]  OutMax=[]  OutDataType=fixdt(1, 16)  ConRadixGroup=Use specified scaling  OutScaling=2^0  OutDataTypeStr=Inherit: Inherit from 'Constant value'
  Constant5 : BaseOperationLib_Browser/Sources&Sinks/Constant  Value=uint8(MCUCoolReqTyp.MCU_NormFlowReq)  OutMin=[]  OutMax=[]  OutDataType=fixdt(1, 16)  ConRadixGroup=Use specified scaling  OutScaling=2^0  OutDataTypeStr=Inherit: Inherit from 'Constant value'
  Constant6 : BaseOperationLib_Browser/Sources&Sinks/Constant  Value=pTMCA_pct_MotWtrPmpNormSpd_C  OutMin=[]  OutMax=[]  OutDataType=fixdt(1, 16)  ConRadixGroup=Use specified scaling  OutScaling=2^0  OutDataTypeStr=Inherit: Inherit from 'Constant value'
  Relational Operator : BaseOperationLib_Browser/Logic Operations Changed/Relational Operator  Operator===  InputSameDT=on  LogicOutDataTypeMode=Specify via dialog  LogicDataType=PDT_Bool  OutDataTypeStr=PDT_Bool
  Relational Operator1 : BaseOperationLib_Browser/Logic Operations Changed/Relational Operator  Operator===  InputSameDT=on  LogicOutDataTypeMode=Specify via dialog  LogicDataType=PDT_Bool  OutDataTypeStr=PDT_Bool
  Relational Operator3 : BaseOperationLib_Browser/Logic Operations Changed/Relational Operator  Operator===  InputSameDT=on  LogicOutDataTypeMode=Specify via dialog  LogicDataType=PDT_Bool  OutDataTypeStr=PDT_Bool
  Switch : BaseOperationLib_Browser/Signal Routing Changed/Switch  Criteria=u2 ~= 0  Threshold=1  InputSameDT=on  OutMin=[]  OutMax=[]  OutDataType=fixdt(1,16,0)  OutScaling=[]  SaturateOnIntegerOverflow=on
  Switch1 : BaseOperationLib_Browser/Signal Routing Changed/Switch  Criteria=u2 ~= 0  Threshold=1  InputSameDT=on  OutMin=[]  OutMax=[]  OutDataType=fixdt(1,16,0)  OutScaling=[]  SaturateOnIntegerOverflow=on
  Switch2 : BaseOperationLib_Browser/Signal Routing Changed/Switch  Criteria=u2 ~= 0  Threshold=1  InputSameDT=on  OutMin=[]  OutMax=[]  OutDataType=fixdt(1,16,0)  OutScaling=[]  SaturateOnIntegerOverflow=on
  pct_Mot1WtrPmpCmd : Outport
  wires:
  Constant2/1 -> Switch1/3
  Switch1/1 -> Switch2/3
  Constant6/1 -> Switch2/1
  Relational Operator3/1 -> Switch2/2
  Constant5/1 -> Relational Operator3/2
  Switch2/1 -> Switch/3
  Switch/1 -> pct_Mot1WtrPmpCmd/1
  Constant4/1 -> Switch1/1
  Relational Operator1/1 -> Switch1/2
  Constant1/1 -> Relational Operator1/2
  Constant3/1 -> Switch/1
  Relational Operator/1 -> Switch/2
  st_MCU1CoolingRequest/1 -> Relational Operator3/1, Relational Operator1/1, Relational Operator/1
  Constant/1 -> Relational Operator/2

== system TMCA_lib/TMCA/Algo/MotorCoolingLoopControl/CoolingPmpControl/MCU2CoolReqProc ==
  st_MCU2CoolingRequest : Inport  OutDataType=fixdt(1, 16)  OutScaling=2^0
  Constant : BaseOperationLib_Browser/Sources&Sinks/Constant  Value=uint8(MCUCoolReqTyp.MCU_MaxFlowReq)  OutMin=[]  OutMax=[]  OutDataType=fixdt(1, 16)  ConRadixGroup=Use specified scaling  OutScaling=2^0  OutDataTypeStr=Inherit: Inherit from 'Constant value'
  Constant1 : BaseOperationLib_Browser/Sources&Sinks/Constant  Value=uint8(MCUCoolReqTyp.MCU_MinFlowReq)  OutMin=[]  OutMax=[]  OutDataType=fixdt(1, 16)  ConRadixGroup=Use specified scaling  OutScaling=2^0  OutDataTypeStr=Inherit: Inherit from 'Constant value'
  Constant2 : BaseOperationLib_Browser/Sources&Sinks/Constant  Value=pTMCA_pct_MotWtrPmpZeroSpd_C  OutMin=[]  OutMax=[]  OutDataType=fixdt(1, 16)  ConRadixGroup=Use specified scaling  OutScaling=2^0  OutDataTypeStr=Inherit: Inherit from 'Constant value'
  Constant3 : BaseOperationLib_Browser/Sources&Sinks/Constant  Value=pTMCA_pct_MotWtrPmpMaxSpd_C  OutMin=[]  OutMax=[]  OutDataType=fixdt(1, 16)  ConRadixGroup=Use specified scaling  OutScaling=2^0  OutDataTypeStr=Inherit: Inherit from 'Constant value'
  Constant4 : BaseOperationLib_Browser/Sources&Sinks/Constant  Value=pTMCA_pct_MotWtrPmpMinSpd_C  OutMin=[]  OutMax=[]  OutDataType=fixdt(1, 16)  ConRadixGroup=Use specified scaling  OutScaling=2^0  OutDataTypeStr=Inherit: Inherit from 'Constant value'
  Constant5 : BaseOperationLib_Browser/Sources&Sinks/Constant  Value=uint8(MCUCoolReqTyp.MCU_NormFlowReq)  OutMin=[]  OutMax=[]  OutDataType=fixdt(1, 16)  ConRadixGroup=Use specified scaling  OutScaling=2^0  OutDataTypeStr=Inherit: Inherit from 'Constant value'
  Constant6 : BaseOperationLib_Browser/Sources&Sinks/Constant  Value=pTMCA_pct_MotWtrPmpNormSpd_C  OutMin=[]  OutMax=[]  OutDataType=fixdt(1, 16)  ConRadixGroup=Use specified scaling  OutScaling=2^0  OutDataTypeStr=Inherit: Inherit from 'Constant value'
  Relational Operator : BaseOperationLib_Browser/Logic Operations Changed/Relational Operator  Operator===  InputSameDT=on  LogicOutDataTypeMode=Specify via dialog  LogicDataType=PDT_Bool  OutDataTypeStr=PDT_Bool
  Relational Operator1 : BaseOperationLib_Browser/Logic Operations Changed/Relational Operator  Operator===  InputSameDT=on  LogicOutDataTypeMode=Specify via dialog  LogicDataType=PDT_Bool  OutDataTypeStr=PDT_Bool
  Relational Operator3 : BaseOperationLib_Browser/Logic Operations Changed/Relational Operator  Operator===  InputSameDT=on  LogicOutDataTypeMode=Specify via dialog  LogicDataType=PDT_Bool  OutDataTypeStr=PDT_Bool
  Switch : BaseOperationLib_Browser/Signal Routing Changed/Switch  Criteria=u2 ~= 0  Threshold=1  InputSameDT=on  OutMin=[]  OutMax=[]  OutDataType=fixdt(1,16,0)  OutScaling=[]  SaturateOnIntegerOverflow=on
  Switch1 : BaseOperationLib_Browser/Signal Routing Changed/Switch  Criteria=u2 ~= 0  Threshold=1  InputSameDT=on  OutMin=[]  OutMax=[]  OutDataType=fixdt(1,16,0)  OutScaling=[]  SaturateOnIntegerOverflow=on
  Switch2 : BaseOperationLib_Browser/Signal Routing Changed/Switch  Criteria=u2 ~= 0  Threshold=1  InputSameDT=on  OutMin=[]  OutMax=[]  OutDataType=fixdt(1,16,0)  OutScaling=[]  SaturateOnIntegerOverflow=on
  pct_Mot2WtrPmpCmd : Outport
  wires:
  Constant/1 -> Relational Operator/2
  st_MCU2CoolingRequest/1 -> Relational Operator/1, Relational Operator1/1, Relational Operator3/1
  Relational Operator/1 -> Switch/2
  Constant3/1 -> Switch/1
  Constant1/1 -> Relational Operator1/2
  Relational Operator1/1 -> Switch1/2
  Constant4/1 -> Switch1/1
  Switch/1 -> pct_Mot2WtrPmpCmd/1
  Switch2/1 -> Switch/3
  Constant5/1 -> Relational Operator3/2
  Relational Operator3/1 -> Switch2/2
  Constant6/1 -> Switch2/1
  Switch1/1 -> Switch2/3
  Constant2/1 -> Switch1/3

== stateflow chart TMCA/Algo/BatteryThermLoopControl/BatHeatingCtrl/Chart ==
  state init
    en:
    time=0;
  state TimeCounter
    en:
    time++;
    du:
    time++;
  (default) -> init
  init -> TimeCounter : [bool_PtcPwrEnbl==1]
  TimeCounter -> init : [bool_PtcPwrEnbl==0]
  data: bool_PtcPwrEnbl input double; time output single

== stateflow chart TMCA/Algo/Task_Flg/Chart1 ==
  state DisEnbl
    en:bool_TMCoolTaskFlg=False;
  state Enbl
    en:bool_TMCoolTaskFlg=True;
  (default) -> DisEnbl
  DisEnbl -> Enbl : [bool_EnblFlg==True]
  Enbl -> DisEnbl : [bool_DisEnblFlg==True]
  data: bool_EnblFlg input double; bool_DisEnblFlg input double; True input double; False input double; bool_TMCoolTaskFlg output boolean

== stateflow chart TMCA/Algo/AC_FAW/Chart ==
  state LvPwrOff
    en:
    bool_IGOffReq = true;
    bool_ACOn = false;
    st_ACMode = ACCtrlModTyp.ACCtrl_ShutDown;
  state LvPwrOn
    en:
    bool_IGOffReq=false;
    bool_ACOn=false;
    bool_VechPermit=true;
    st_ACMode = ACCtrlModTyp.ACCtrl_INIT;
  state HvPwrOn
    en:
    bool_IGOffReq=false;
    bool_ACOn=true;
    st_ACMode = ACCtrlModTyp.ACCtrl_HvPwrOn;
    state DisChrgJudge
      en:
      bool_ACOn=true;
    state ACON
      en:
      bool_ACOn=true;
    state ACOFF
      en:
      bool_ACOn=false;
    (default) -> ACON
    ACON -> DisChrgJudge : [A_BatCurr>=A_BatCurrHi &&...
        | (st_PUDCoorrSts==PUDCoorrStsTyp.PUD_ACChrgOn||...
        | st_PUDCoorrSts==PUDCoorrStsTyp.PUD_DCChrgOn||...
        | st_PUDCoorrSts==PUDCoorrStsTyp.PUD_ACHeatOn||...
        | st_PUDCoorrSts==PUDCoorrStsTyp.PUD_DCHeatOn)]
    DisChrgJudge -> ACON [order 1] : [A_BatCurr<=A_BatCurrLo]
    DisChrgJudge -> ACOFF [order 2] : after(pTMCA_s_ACDisChrgTimout_C,sec)
  LvPwrOff -> LvPwrOn : [st_PUDCoorrSts != PUDCoorrStsTyp.PUD_EmgHVOFF_OK && ...
      | st_PUDCoorrSts != PUDCoorrStsTyp.PUD_HVOFF_OK]
  LvPwrOn -> LvPwrOff [order 2] : [st_PUDCoorrSts == PUDCoorrStsTyp.PUD_EmgHVOFF_OK || ...
      | st_PUDCoorrSts == PUDCoorrStsTyp.PUD_HVOFF_OK]
  (default) -> LvPwrOn
  LvPwrOn -> HvPwrOn [order 1] : [bool_AcPwrEnbl == true]
  HvPwrOn -> LvPwrOn : [bool_AcPwrEnbl == false]
  data: bool_VechPermit output boolean; bool_IGOffReq output boolean; bool_ACOn output boolean; st_ACMode output uint8; bool_AcPwrEnbl input double; st_PUDCoorrSts input double; A_BatCurr input double; bool_BatCoolgReq input double; pTMCA_s_ACDisChrgTimout_C input double; A_BatCurrHi input double; A_BatCurrLo input double

== stateflow chart TMCA/Algo/Task_Flg/Chart ==
  state DisEnbl
    en:bool_TMCoolTaskFlg=False;
  state Enbl
    en:bool_TMCoolTaskFlg=True;
  (default) -> DisEnbl
  DisEnbl -> Enbl : [bool_EnblFlg==True]
  Enbl -> DisEnbl : [bool_DisEnblFlg==True]
  data: bool_EnblFlg input double; bool_DisEnblFlg input double; True input double; False input double; bool_TMCoolTaskFlg output boolean
